simulink model "statelessWriter2_1"  (Simulink 9.3)
settings: Solver=VariableStepAuto  StartTime=0.0  StopTime=10.0  RelTol=1e-3
settings Model: Creator=root  LastModifiedBy=BEAR
settings DataIOCC: SaveFormat=Dataset  SignalLoggingSaveFormat=Dataset
settings OptimizationCC: LifeSpan=auto
settings DebuggingCC: UnderspecifiedInitializationDetection=Simplified  MergeDetectMultiDrivingBlocksExec=error  FcnCallInpInsideContextMsg=error  SFUnexpectedBacktrackingDiag=error  SFNoUnconditionalDefaultTransitionDiag=error  SFExecutionAtInitializationDiag=warning
settings HardwareCC: ProdBitPerPointer=64  ProdBitPerSizeT=64  ProdBitPerPtrDiffT=64  ProdLargestAtomicFloat=Float  ProdIntDivRoundTo=Zero  ProdEndianess=LittleEndian  ProdWordSize=64  ProdHWDeviceType=Intel->x86-64 (Windows64)
settings ModelReferenceCC: PropagateSignalLabelsOutOfModel=on
settings GRTTargetCC: TargetLangStandard=C99 (ISO)  CombineOutputUpdateFcns=on  GRTInterface=off
settings ConfigComp: CovMetricSettings=dwe  CovHtmlReporting=off  CovSaveCumulativeToWorkspaceVar=off  CovSaveSingleToWorkspaceVar=off  CovExternalEMLEnable=on

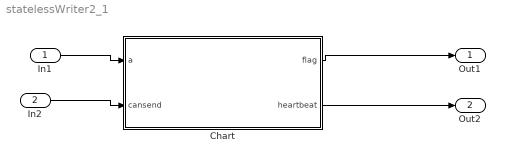
== system statelessWriter2_1 ==
  In1 : Inport
  In2 : Inport  Port=2
  Chart : Stateflow chart  TreatAsAtomicUnit=on
  Out1 : Outport
  Out2 : Outport  Port=2
  wires:
  In1/1 -> Chart/1(a)
  In2/1 -> Chart/2(cansend)
  Chart/1(flag) -> Out1/1
  Chart/2(heartbeat) -> Out2/1

== stateflow chart Chart ==
  settings: updateMethod=DISCRETE  sampleTime=0.01
  state pushing
    during:flag=0
  state idle
    entry:heartbeat=0;
    during:flag=1;
  note: [cansend==1]/{i=i-1}
  (default) -> idle : {i=a}
  pushing -> pushing [order 2]
  pushing -> idle [order 1] : [i<=0]
  idle -> pushing [order 1] : [i>0]
  idle -> idle [order 2] : after(heartbeatPeriod,sec){heartbeat=1}
  data: a input double; i local double; flag output double; cansend input double; heartbeatPeriod constant double; heartbeat output double
  events: event local FUNCTION_CALL_EVENT; event1 local FUNCTION_CALL_EVENT
